simulink model "sim_pos_att1"  (R2018b)
settings: Solver=ode1  StartTime=0.0  StopTime=20  FixedStep=dt  RelTol=1e-3
undefined symbols (not defined in the file or in its folder): GRAVITY_MSS, gyro_x, gyro_y, gyro_z, HD, Kd, Ku, Ld, Ldx, Ldy, Lu, Lux, Luy, m, p_angle_pitch, p_angle_yaw, pwm_max, pwm_min, Qd, Qu
libraries: shared6dof x1
(part 2 of 2)

== matlab function sim_pos_att1/MATLAB Function ==
  settings: updateMethod=DISCRETE
  data: pwm_out input; F output; gn input; M output; Ku parameter; Kd parameter; Lux parameter; Luy parameter; Ldx parameter; Ldy parameter; Lu parameter; Ld parameter; pwm_min parameter; pwm_max parameter; Qu parameter; Qd parameter
function [F ,M] = mode_F_M(pwm_out, gn, Ku, Kd, Lux, Luy, Ldx, Ldy, Lu, Ld, pwm_min, pwm_max, Qu, Qd)
% global pwm_min
% global pwm_max
% global Ku
% global Kd
% global Lux
% global Luy
% global Ldx
% global Ldy
% global Lu
% global Ld
F1=(pwm_out(1)-pwm_min)/(pwm_max-pwm_min)*Ku;
F2=(pwm_out(2)-pwm_min)/(pwm_max-pwm_min)*Kd;
F3=(pwm_out(3)-pwm_min)/(pwm_max-pwm_min)*Ku;
F4=(pwm_out(4)-pwm_min)/(pwm_max-pwm_min)*Kd;


F=-[0 0 F1+F2+F3+F4]'+gn;
Mx=(-F1+F3)*Lux+(F2-F4)*Ldx;
My=(F1+F3)*Luy+(-F2-F4)*Ldy;
Mz=(-F1+F3)*Lu*sind(Qu)+(-F2+F4)*Ld*sind(Qd);%0.1736=sind(10)  0.1071= Ld*900*sind(10)/(Lu*1600)
M=[Mx My Mz];
end

== matlab function sim_pos_att1/update_z_controller ==
  data: recalc_leash_z data_store_memory; leash_up_z data_store_memory; POSCONTROL_SPEED_UP data_store_memory; POSCONTROL_ACCEL_Z data_store_memory; POSCONTROL_POS_Z_P data_store_memory; leash_down_z data_store_memory; POSCONTROL_SPEED_DOWN data_store_memory; POSCONTROL_ACCELERATION_MIN data_store_memory; POSCONTROL_LEASH_LENGTH_MIN data_store_memory; limit_pos_up data_store_memory; limit_pos_down data_store_memory; pos_error data_store_memory; pos_target data_store_memory; curr_alt data_store_memory; vel_target data_store_memory; dt data_store_memory; limit_vel_up data_store_memory; limit_vel_down data_store_memory; use_desvel_ff_z data_store_memory; reset_rate_to_accel_z data_store_memory; vel_desired data_store_memory; accel_desired data_store_memory; POSCONTROL_VEL_ERROR_CUTOFF_FREQ data_store_memory; vel_last data_store_memory; freeze_ff_z data_store_memory; vel_error data_store_memory; vel_error_input data_store_memory; curr_vel data_store_memory; accel_target data_store_memory; POSCONTROL_VEL_Z_P data_store_memory; reset_accel_to_throttle data_store_memory; accel_error data_store_memory; z_accel_meas data_store_memory; pid_accel_z_reset_filter data_store_memory; POSCONTROL_ACC_Z_FILT_HZ data_store_memory; pid_accel_z_input data_store_memory; pid_accel_z_derivative data_store_memory; POSCONTROL_ACC_Z_P data_store_memory; pid_accel_z_integrator data_store_memory; POSCONTROL_ACC_Z_IMAX data_store_memory; throttle_hover data_store_memory; throttle_lower data_store_memory; throttle_upper data_store_memory; POSCONTROL_ACC_Z_D data_store_memory; throttle_input data_store_memory; POSCONTROL_ACC_Z_I data_store_memory; throttle_thrust_max data_store_memory; althold_lean_angle_max data_store_memory; angle_limit_tc data_store_memory; angle_boost_enabled data_store_memory; pitch data_store_memory; roll data_store_memory; angle_boost data_store_memory; throttle_rpy_mix data_store_memory; throttle_avg_max data_store_memory; AC_ATTITUDE_CONTROL_ANGLE_LIMIT_THROTTLE_MAX data_store_memory; POSCONTROL_POS_XY_P data_store_memory; curr_pos data_store_memory; leash data_store_memory; POSCONTROL_ACCEL_XY data_store_memory; POSCONTROL_VEL_XY_FILT_HZ data_store_memory; POSCONTROL_VEL_XY_FILT_D_HZ data_store_memory; pid_vel_xy_reset_filter data_store_memory; pid_vel_xy_input data_store_memory; pid_vel_xy_derivative data_store_memory; pid_vel_xy_integrator data_store_memory; POSCONTROL_VEL_XY_P data_store_memory; limit_accel_xy data_store_memory; motors_limit_throttle_upper data_store_memory; POSCONTROL_VEL_XY_I data_store_memory; POSCONTROL_VEL_XY_IMAX data_store_memory; POSCONTROL_VEL_XY_D data_store_memory; reset_accel_to_lean_xy data_store_memory; POSCONTROL_ACCEL_FILTER_HZ data_store_memory; accel_xy_input data_store_memory; accel_xy_angle_max data_store_memory; roll_target data_store_memory; pitch_target data_store_memory; GRAVITY_MSS data_store_memory; POSCONTROL_ACCEL_XY_MAX data_store_memory; yaw data_store_memory; recalc_leash_xy data_store_memory; POSCONTROL_SPEED data_store_memory; reset_desired_vel_to_pos data_store_memory; POSCONTROL_OVERSPEED_GAIN_Z data_store_memory; POSCONTROL_JERK_RATIO data_store_memory; accel_last_z_cms data_store_memory; is_active_z data_store_memory; POSCONTROL_STOPPING_DIST_DOWN_MAX data_store_memory; POSCONTROL_STOPPING_DIST_UP_MAX data_store_memory; is_active_xy data_store_memory; rot_body_to_ned data_store_memory; attitude_target_quat data_store_memory; attitude_target_ang_vel data_store_memory; thrust_error_angle data_store_memory; rate_target_ang_vel data_store_memory; gyro_z data_store_memory; ang_vel_roll_max data_store_memory; ang_vel_pitch_max data_store_memory; ang_vel_yaw_max data_store_memory; AC_ATTITUDE_THRUST_ERROR_ANGLE data_store_memory; rate_bf_ff_enabled data_store_memory; attitude_ang_error data_store_memory; p_angle_yaw data_store_memory; AC_ATTITUDE_ACCEL_Y_CONTROLLER_MAX_RADSS data_store_memory; use_sqrt_controller data_store_memory; p_angle_roll data_store_memory; AC_ATTITUDE_ACCEL_RP_CONTROLLER_MIN_RADSS data_store_memory; AC_ATTITUDE_ACCEL_RP_CONTROLLER_MAX_RADSS data_store_memory; p_angle_pitch data_store_memory; accel_pitch_max data_store_memory; accel_yaw_max data_store_memory; accel_roll_max data_store_memory; AC_ATTITUDE_ACCEL_Y_CONTROLLER_MIN_RADSS data_store_memory; attitude_target_euler_angle data_store_memory; input_tc data_store_memory; attitude_target_euler_rate data_store_memory; slew_yaw data_store_memory; rate_pitch_pid_reset_filter data_store_memory; rate_pitch_pid_input data_store_memory; rate_pitch_pid_derivative data_store_memory; rate_pitch_pid_integrator data_store_memory; motors_limit_roll_pitch data_store_memory; ATC_RAT_PIT_D data_store_memory; ATC_RAT_PIT_FF data_store_memory; ATC_RAT_PIT_FILT data_store_memory; ATC_RAT_PIT_I data_store_memory; ATC_RAT_PIT_IMAX data_store_memory; ATC_RAT_PIT_P data_store_memory; ATC_RAT_RLL_D data_store_memory; ATC_RAT_RLL_FF data_store_memory; ATC_RAT_RLL_FILT data_store_memory; ATC_RAT_RLL_I data_store_memory; ATC_RAT_RLL_IMAX data_store_memory; ATC_RAT_RLL_P data_store_memory; rate_roll_pid_reset_filter data_store_memory; rate_roll_pid_input data_store_memory; rate_roll_pid_derivative data_store_memory; rate_roll_pid_integrator data_store_memory; ATC_RAT_YAW_D data_store_memory; ATC_RAT_YAW_FF data_store_memory; ATC_RAT_YAW_FILT data_store_memory; ATC_RAT_YAW_I data_store_memory; ATC_RAT_YAW_IMAX data_store_memory; ATC_RAT_YAW_P data_store_memory; rate_yaw_pid_reset_filter data_store_memory; rate_yaw_pid_input data_store_memory; rate_yaw_pid_derivative data_store_memory; rate_yaw_pid_integrator data_store_memory; motors_limit_yaw data_store_memory; gyro_x data_store_memory; gyro_y data_store_memory; inint data_store_memory; AP_MOTORS_MATRIX_YAW_FACTOR_CCW data_store_memory; AP_MOTORS_MATRIX_YAW_FACTOR_CW data_store_memory; pitch_factor data_store_memory; roll_factor data_store_memory; yaw_factor data_store_memory; throttle_in data_store_memory; throttle_cutoff_frequency data_store_memory; POSCONTROL_THROTTLE_CUTOFF_FREQ data_store_memory; throttle_filter data_store_memory; armed data_store_memory; roll_in data_store_memory; pitch_in data_store_memory; yaw_in data_store_memory; thrust_boost_ratio data_store_memory; thrust_rpyt_out data_store_memory; limit_roll_pitch data_store_memory; yaw_headroom data_store_memory; thrust_boost data_store_memory; limit_yaw data_store_memory; current_tilt data_store_memory; air_density_ratio data_store_memory; pwm_max data_store_memory; pwm_min data_store_memory; thrust_slew_time data_store_memory; pwm_out data_store_memory; attitude_error_vector data_store_memory; mode_fy data_store_memory
function update_vel_controller_xyz

global rate_target_ang_vel
global gyro_x
global gyro_y
global gyro_z
global roll_target
global pitch_target
global roll_in
global pitch_in
global yaw_in
global inint
    if(inint)
    setup_motors() ;
    inint=0;
    end
update_vel_controller_xyz()
% input_euler_angle_roll_pitch_euler_rate_yaw(  roll_target,   pitch_target,   0)
input_euler_angle_roll_pitch_euler_rate_yaw(  roll_target,   pitch_target,   0)

roll_in=rate_target_to_motor_roll(  gyro_x,  rate_target_ang_vel(1));
pitch_in=rate_target_to_motor_pitch( gyro_y,  rate_target_ang_vel(2));
yaw_in=rate_target_to_motor_yaw(  gyro_z,   rate_target_ang_vel(3));

% roll_in=rate_target_to_motor_roll(  gyro_x,  0);
% pitch_in=rate_target_to_motor_pitch( gyro_y,  0);
% yaw_in=rate_target_to_motor_yaw(  gyro_z,   0.1);

AP_MotorsMulticopter_output()
end

== matlab function sim_pos_att1/MATLAB Function1 ==
  data: q input; euler_angle output
function euler_angle= to_euler(q)

euler_angle= to_euler(q);

== matlab function sim_pos_att1/MATLAB Function2 ==
  data: q input; euler_angle output
function euler_angle= to_euler(q)

euler_angle= to_euler(q);
